simulink model "EBike_Braking"  (R2019b)
settings: Solver=VariableStepAuto  StartTime=0.0  StopTime=1000  MaxStep=0.01  RelTol=1e-3
values from neighbouring files (symbols this model uses):
  A_d = 0.4    [Thesis_Ebike.m]
  Abs = 1    [Thesis_Ebike.m]
  alpha_Conductor = 0.0040    (= 0.004)    [Thesis_Ebike.m]
  Alpha_Magnet = -0.0020    (= -0.002)    [Thesis_Ebike.m]
  Bm = ((Motor_torque_constant)*(17)/(1000*2*pi/60))    (= 0.121753531465)    [Thesis_Ebike.m]
  Braking_Pressure = 100    [Thesis_Ebike.m]
  C_d = 0.9    [Thesis_Ebike.m]
  capacity = 19.5    [Thesis_Ebike.m]
  Coefficient_of_Brake_friction = 0.9    [Thesis_Ebike.m]
  Crank_Length = 0.150    (= 0.15)    [Thesis_Ebike.m]
  Cyclist_weight = 85    [Thesis_Ebike.m]
  Dynamic_Friction_Coefficient = 0.0015    [Thesis_Ebike.m]
  Effective_Radius_of_Disc = 0.16    [Thesis_Ebike.m]
  F_Rider = 100    [Thesis_Ebike.m]
  g = 9.81    [Thesis_Ebike.m]
  Internal_Resistance = 95*10^-3    (= 0.095)    [Thesis_Ebike.m]
  Jm = 10.2 *10^-3    (= 0.0102)    [Thesis_Ebike.m]
  Kb = (51.7/(1000*2*pi/60))    (= 0.493698633471)    [Thesis_Ebike.m]
  L = 0.36*10^-3    (= 0.00036)    [Thesis_Ebike.m]
  Motor_resistance = 88*10^-2    (= 0.88)    [Thesis_Ebike.m]
  Motor_torque_constant = 0.75    [Thesis_Ebike.m]
  Polarization_Capacitance = 1*10^-7    (= 1e-07)    [Thesis_Ebike.m]
  Polarization_Resistance = 95*10^-3    (= 0.095)    [Thesis_Ebike.m]
  Ref_Temp = 25    [Thesis_Ebike.m]
  Rho_air = 1.225    [Thesis_Ebike.m]
  SOC_initial = 100    [Thesis_Ebike.m]
  Static_Friction_Coefficient = 0.0015    [Thesis_Ebike.m]
  Tire_mass = 0.25    [Thesis_Ebike.m]
  Trailer_mass = 50    [Thesis_Ebike.m]
  Vehicle_mass = 25    [Thesis_Ebike.m]
  Wheel_Inertia = 0.0225    [Thesis_Ebike.m]
  Wheel_mass = 0.25    [Thesis_Ebike.m]
  Wheel_Radius = 0.3    [Thesis_Ebike.m]
undefined symbols (not defined in the file or in its folder): sigbuilder_block, V
libraries: simulink x2
(part 1 of 3)
settings Model: Creator=Avmash  LastModifiedBy=Avmash
settings SolverCC: ZeroCrossAlgorithm=Adaptive
settings DebuggingCC: IgnoredZcDiagnostic=none

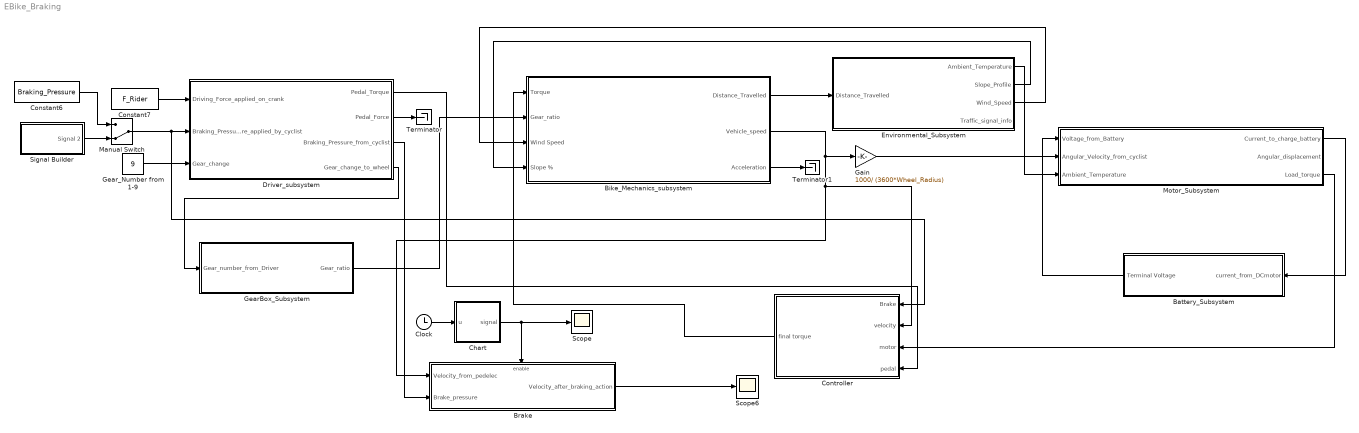
== system EBike_Braking ==
  Battery_Subsystem : Subsystem
  Bike_Mechanics_subsystem : Subsystem
  Brake : Subsystem  TreatAsAtomicUnit=on
  Chart : Stateflow chart  BlockKeywords=__PRM__SERIALIZED__DATA__:Stateflow Chart,Stateflow Diagram  TreatAsAtomicUnit=on
  Clock : Clock
  Constant6 : Constant  Value=Braking_Pressure
  Constant7 : Constant  Value=F_Rider
  Controller : Subsystem
  Driver_subsystem : Subsystem
  Environmental_Subsystem : Subsystem
  Gain : Gain  Gain=1000/ (3600*Wheel_Radius)
  GearBox_Subsystem : Subsystem
  Gear_Number from 1-9 : Constant  Value=9
  Manual Switch : ManualSwitch  CurrentSetting=0
  Motor_Subsystem : Subsystem
  Scope : Scope
  Scope6 : Scope
  Signal Builder : Subsystem  Tag=STV Subsys  LoadFcn=sigbuilder_block('load');  StartFcn=sigbuilder_block('start');  StopFcn=sigbuilder_block('stop');  ClipboardFcn=sigbuilder_block('clipboard');  mask(Sigbuilder block){tuvar=[0:10]}
      mask help: Simulink:masks:SigbuilderBlock_MD
      mask init:
      | if ~strcmp(get_param(bdroot(gcbh),'SimulationStatus'),'stopped') tuvar = sigbuilder_block('maskInit'); end
      settings: CopyFcn=sigbuilder_block('copy');  DeleteFcn=sigbuilder_block('delete');  ModelCloseFcn=sigbuilder_block('modelClose');  PreSaveFcn=sigbuilder_block('preSave');  PauseFcn=sigbuilder_block('pause');  ContinueFcn=sigbuilder_block('continue');  NameChangeFcn=sigbuilder_block('namechange');  OpenFcn=sigbuilder_block('open',[437.6 153 550.4 359.25 ]);  CloseFcn=sigbuilder_block('close');
      mask Display: plot(0, 0, 100, 100,[2, 2, 32, 32, 2], [68, 8, 8, 68, 68],[32, 2], [38, 38], [32, 19, 2],[53, 60, 44], [32, 17, 17, 2],[16, 16, 31, 31]);txt = getActiveGroup(gcbh);text(2, 100, txt,'verticalAlignment', 'top');
  Terminator : Terminator
  Terminator1 : Terminator
  wires:
  Environmental_Subsystem/2(Slope_Profile) -> Bike_Mechanics_subsystem/4(Slope %)
  Environmental_Subsystem/3(Wind_Speed) -> Bike_Mechanics_subsystem/3(Wind Speed)
  Brake/1(Velocity_after_braking_action) -> Scope6/1
  Manual Switch/1 -> Controller/1(Brake), Driver_subsystem/2(Braking_Pressure_applied_by_cyclist)
  Signal Builder/1(Signal 2) -> Manual Switch/2
  Driver_subsystem/3(Braking_Pressure_from_cyclist) -> Brake/2(Brake_pressure)
  Constant6/1 -> Manual Switch/1
  Clock/1 -> Chart/1(u)
  Controller/1("final torque ") -> Bike_Mechanics_subsystem/1(Torque)
  Bike_Mechanics_subsystem/1(Distance_Travelled) -> Environmental_Subsystem/1(Distance_Travelled)
  Chart/1(signal) -> Scope/1, Brake/Enable
  Environmental_Subsystem/1(Ambient_Temperature) -> Motor_Subsystem/3(Ambient_Temperature)
  Gain/1 -> Motor_Subsystem/2(Angular_Velocity_from_cyclist)
  Driver_subsystem/4(Gear_change_to_wheel) -> GearBox_Subsystem/1(Gear_number_from_Driver)
  Bike_Mechanics_subsystem/2(Vehicle_speed) -> Brake/1(Velocity_from_pedelec), Controller/2(velocity), Gain/1
  Motor_Subsystem/1(Current_to_charge_battery) -> Battery_Subsystem/1(current_from_DCmotor)
  Driver_subsystem/1(Pedal_Torque) -> Controller/4(pedal)
  Driver_subsystem/2(Pedal_Force) -> Terminator/1
  GearBox_Subsystem/1(Gear_ratio) -> Bike_Mechanics_subsystem/2(Gear_ratio)
  Constant7/1 -> Driver_subsystem/1(Driving_Force_applied_on_crank)
  Gear_Number from 1-9/1 -> Driver_subsystem/3(Gear_change)
  Motor_Subsystem/3(Load_torque) -> Controller/3(motor)
  Battery_Subsystem/1(Terminal Voltage) -> Motor_Subsystem/1(Voltage_from_Battery)
  Bike_Mechanics_subsystem/3(Acceleration) -> Terminator1/1

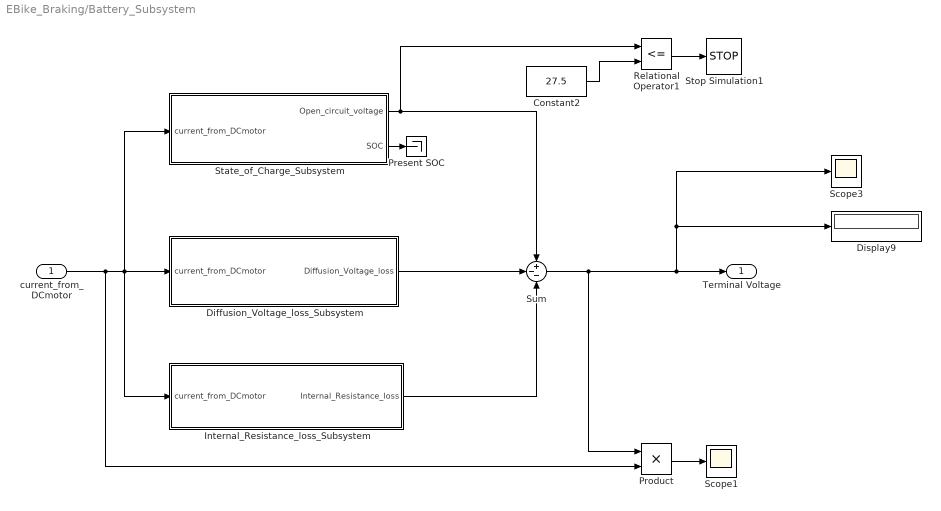
== system EBike_Braking/Battery_Subsystem ==
  current_from_DCmotor : Inport
  Constant2 : Constant  Value=27.5
  Diffusion_Voltage_loss_Subsystem : Subsystem
  Display9 : Display
  Internal_Resistance_loss_Subsystem : Subsystem
  Present SOC : Terminator
  Product : Product
  Relational Operator1 : RelationalOperator  Operator=<=  OutDataTypeStr=boolean  RndMeth=Simplest
  Scope1 : Scope
  Scope3 : Scope
  "State_of_Charge_Subsystem " : Subsystem
  Stop Simulation1 : Stop
  Sum : Sum  Inputs=+--
  Terminal Voltage : Outport  VectorParamsAs1DForOutWhenUnconnected=off
  wires:
  current_from_DCmotor/1 -> Product/2, Internal_Resistance_loss_Subsystem/1(current_from_DCmotor), "State_of_Charge_Subsystem "/1(current_from_DCmotor), Diffusion_Voltage_loss_Subsystem/1(current_from_DCmotor)
  "State_of_Charge_Subsystem "/2(SOC) -> Present SOC/1
  Relational Operator1/1 -> Stop Simulation1/1
  Constant2/1 -> Relational Operator1/2
  Internal_Resistance_loss_Subsystem/1(Internal_Resistance_loss) -> Sum/3
  Diffusion_Voltage_loss_Subsystem/1(Diffusion_Voltage_loss) -> Sum/2
  "State_of_Charge_Subsystem "/1(Open_circuit_voltage) -> Sum/1, Relational Operator1/1
  Sum/1 -> Product/1, Display9/1, Scope3/1, Terminal Voltage/1
  Product/1 -> Scope1/1

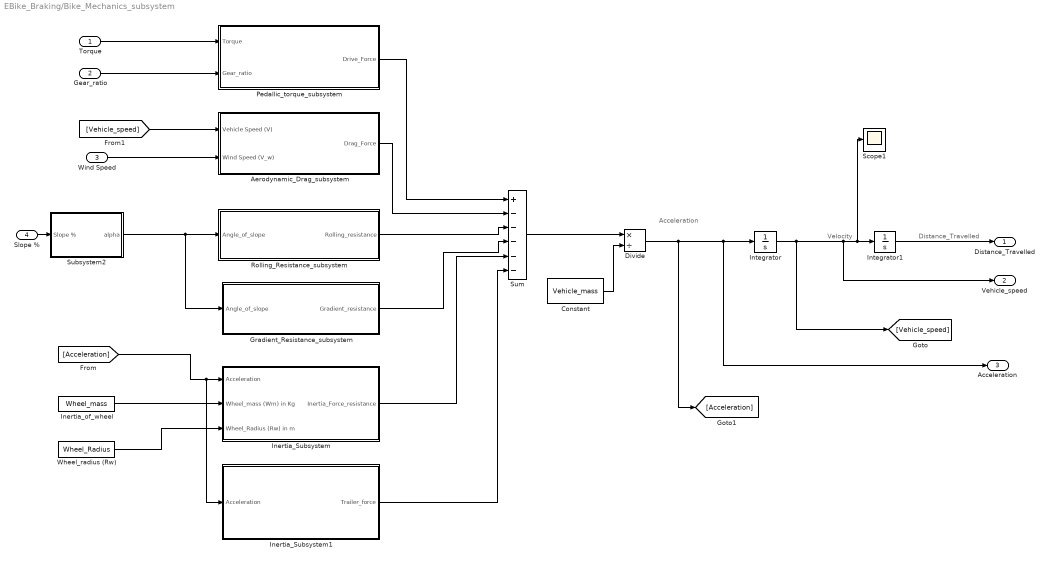
== system EBike_Braking/Bike_Mechanics_subsystem ==
  note: Acceleration
  note: Velocity
  note: Distance_Travelled
  Torque : Inport
  Gear_ratio : Inport  Port=2
  Wind Speed : Inport  Port=3
  Slope % : Inport  Port=4
  Aerodynamic_Drag_subsystem : Subsystem
  Constant : Constant  Value=Vehicle_mass  SampleTime=-1
  Divide : Product  Inputs=*/
  Gradient_Resistance_subsystem : Subsystem
  Inertia_Subsystem : Subsystem
  Inertia_Subsystem1 : Subsystem
  Inertia_of_wheel : Constant  Value=Wheel_mass
  Integrator : Integrator  LowerSaturationLimit=0
  Integrator1 : Integrator
  Pedallic_torque_subsystem : Subsystem
  Rolling_Resistance_subsystem : Subsystem
  Scope1 : Scope
  Subsystem2 : Subsystem
  Sum : Sum  Inputs=+-----
  "Wheel_radius (Rw) " : Constant  Value=Wheel_Radius
  Distance_Travelled : Outport  VectorParamsAs1DForOutWhenUnconnected=off
  Vehicle_speed : Outport  Port=2  VectorParamsAs1DForOutWhenUnconnected=off
  Acceleration : Outport  Port=3  VectorParamsAs1DForOutWhenUnconnected=off
  wires:
  Inertia_Subsystem/1(Inertia_Force_resistance) -> Sum/5
  [Acceleration] -> Inertia_Subsystem1/1(Acceleration), Inertia_Subsystem/1(Acceleration)
  Rolling_Resistance_subsystem/1(Rolling_resistance) -> Sum/3
  "Wheel_radius (Rw) "/1 -> Inertia_Subsystem/3(Wheel_Radius (Rw) in m)
  [Vehicle_speed] -> Aerodynamic_Drag_subsystem/1(Vehicle Speed (V))
  Pedallic_torque_subsystem/1(Drive_Force) -> Sum/1
  Gradient_Resistance_subsystem/1(Gradient_resistance) -> Sum/4
  Wind Speed/1 -> Aerodynamic_Drag_subsystem/2("Wind Speed (V_w) ")
  Aerodynamic_Drag_subsystem/1("Drag_Force ") -> Sum/2
  Inertia_of_wheel/1 -> Inertia_Subsystem/2(Wheel_mass (Wm) in Kg)
  Constant/1 -> Divide/2
  Divide/1 -> Integrator/1, Acceleration/1, [Acceleration]
  Integrator/1 -> [Vehicle_speed], Scope1/1, Integrator1/1, Vehicle_speed/1
  Subsystem2/1(alpha) -> Gradient_Resistance_subsystem/1(Angle_of_slope), Rolling_Resistance_subsystem/1(Angle_of_slope)
  Sum/1 -> Divide/1
  Gear_ratio/1 -> Pedallic_torque_subsystem/2(Gear_ratio)
  Torque/1 -> Pedallic_torque_subsystem/1(Torque)
  Integrator1/1 -> Distance_Travelled/1
  Slope %/1 -> Subsystem2/1(Slope %)
  Inertia_Subsystem1/1(Trailer_force) -> Sum/6

== system EBike_Braking/Brake ==
  Velocity_from_pedelec : Inport
  Brake_pressure : Inport  Port=2
  Enable : EnablePort
  Scope{,1..3} (4 alike) : Scope
  Subsystem1 : Subsystem
  Velocity_after_braking_action : Outport
  wires:
  Subsystem1/2(velocity_of_bike) -> Scope2/1, Velocity_after_braking_action/1
  Velocity_from_pedelec/1 -> Scope/1, Subsystem1/1(velocity)
  Subsystem1/1(Wheel_Velocity) -> Scope1/1
  Subsystem1/3(stopping_distance) -> Scope3/1
  Brake_pressure/1 -> Subsystem1/2(Brake_pressure)

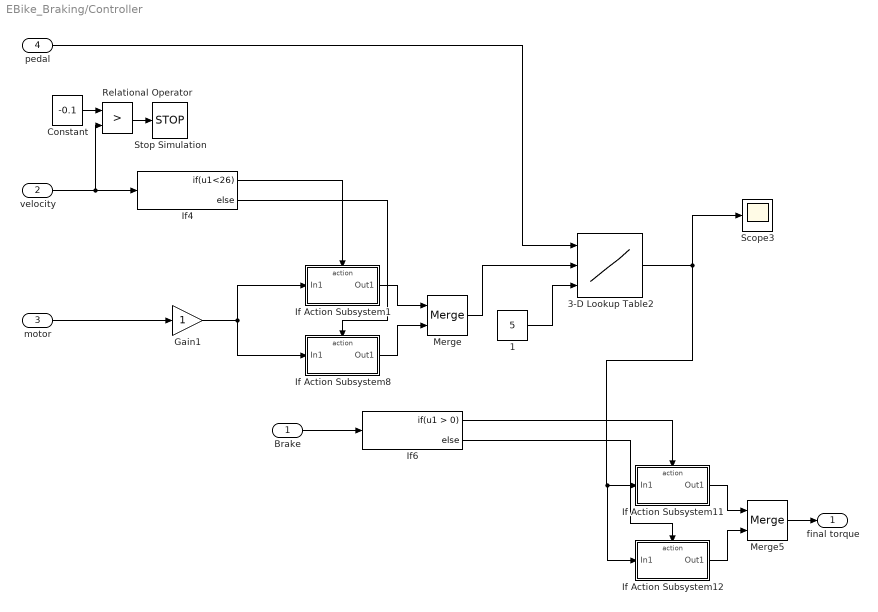
== system EBike_Braking/Controller ==
  Brake : Inport
  velocity : Inport  Port=2
  motor : Inport  Port=3
  pedal : Inport  Port=4
  " 1" : Constant  Value=5
  3-D Lookup Table2 : Lookup_n-D  NumberOfTableDimensions=3  BreakpointsForDimension1=[0,5,10,15,20]  BreakpointsForDimension2=[0,10,20,30,40]  BreakpointsForDimension3=[5, 7]  Table=reshape([0,5,10,15,20,0,10,15,20,25,0,10,20,25,30,0,10,20,30,35,0,10,20,30,40,0,5,10,15,20,0,10,15,20,25,0,10,20,25,30,0,10,20,30,35,0,10,20,30,40],5,5,2)  InternalRulePriority=Speed  RndMeth=Simplest  InputSameDT=on
  Constant : Constant  Value=-0.1
  Gain1 : Gain
  If Action Subsystem1 : Subsystem  TreatAsAtomicUnit=on
  If Action Subsystem11 : Subsystem  TreatAsAtomicUnit=on
  If Action Subsystem12 : Subsystem  TreatAsAtomicUnit=on
  If Action Subsystem8 : Subsystem  TreatAsAtomicUnit=on
  If4 : If  IfExpression=u1<26
  If6 : If
  Merge : Merge
  Merge5 : Merge
  Relational Operator : RelationalOperator  Operator=>  OutDataTypeStr=boolean  RndMeth=Simplest
  Scope3 : Scope
  Stop Simulation : Stop
  "final torque " : Outport
  wires:
  Brake/1 -> If6/1
  If6/2 -> If Action Subsystem12/Action
  If6/1 -> If Action Subsystem11/Action
  If Action Subsystem11/1(Out1) -> Merge5/1
  Merge5/1 -> "final torque "/1
  If Action Subsystem12/1(Out1) -> Merge5/2
  motor/1 -> Gain1/1
  velocity/1 -> Relational Operator/2, If4/1
  " 1"/1 -> 3-D Lookup Table2/3
  If Action Subsystem1/1(Out1) -> Merge/1
  If4/1 -> If Action Subsystem1/Action
  3-D Lookup Table2/1 -> If Action Subsystem12/1(In1), If Action Subsystem11/1(In1), Scope3/1
  Gain1/1 -> If Action Subsystem8/1(In1), If Action Subsystem1/1(In1)
  pedal/1 -> 3-D Lookup Table2/1
  Merge/1 -> 3-D Lookup Table2/2
  If4/2 -> If Action Subsystem8/Action
  If Action Subsystem8/1(Out1) -> Merge/2
  Constant/1 -> Relational Operator/1
  Relational Operator/1 -> Stop Simulation/1

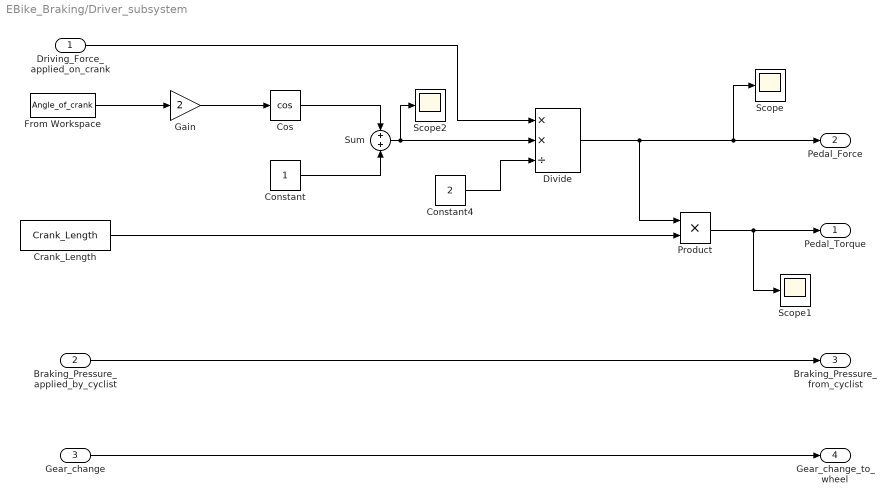
== system EBike_Braking/Driver_subsystem ==
  Driving_Force_applied_on_crank : Inport
  Braking_Pressure_applied_by_cyclist : Inport  Port=2
  Gear_change : Inport  Port=3
  Constant : Constant
  Constant4 : Constant  Value=2
  Cos : Trigonometry  Operator=cos
  Crank_Length : Constant  Value=Crank_Length
  Divide : Product  Inputs=**/
  From Workspace : FromWorkspace  VariableName=Angle_of_crank  SampleTime=0
  Gain : Gain  Gain=2
  Product : Product
  Scope : Scope
  Scope1 : Scope
  Scope2 : Scope
  Sum : Sum
  Pedal_Torque : Outport
  Pedal_Force : Outport  Port=2
  Braking_Pressure_from_cyclist : Outport  Port=3
  Gear_change_to_wheel : Outport  Port=4  VectorParamsAs1DForOutWhenUnconnected=off
  wires:
  Divide/1 -> Scope/1, Pedal_Force/1, Product/1
  Gain/1 -> Cos/1
  Constant/1 -> Sum/2
  Cos/1 -> Sum/1
  Product/1 -> Scope1/1, Pedal_Torque/1
  Constant4/1 -> Divide/3
  Driving_Force_applied_on_crank/1 -> Divide/1
  Sum/1 -> Scope2/1, Divide/2
  Crank_Length/1 -> Product/2
  Braking_Pressure_applied_by_cyclist/1 -> Braking_Pressure_from_cyclist/1
  From Workspace/1 -> Gain/1
  Gear_change/1 -> Gear_change_to_wheel/1

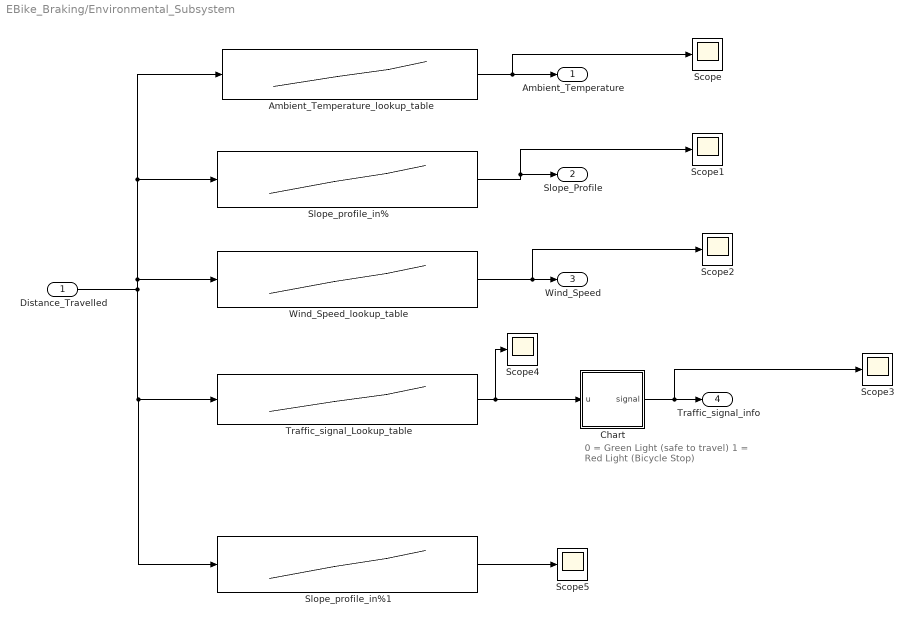
== system EBike_Braking/Environmental_Subsystem ==
  note: 0 = Green Light (safe to travel)
      | 1 = Red Light (Bicycle Stop)
  Distance_Travelled : Inport
  Ambient_Temperature_lookup_table : Lookup_n-D  NumberOfTableDimensions=1  BreakpointsForDimension1=[0 6000 12000]  Table=[25 24 25]  InternalRulePriority=Speed  RndMeth=Simplest  InputSameDT=on
  Chart : Stateflow chart  BlockKeywords=__PRM__SERIALIZED__DATA__:Stateflow Chart,Stateflow Diagram  TreatAsAtomicUnit=on
  Scope{,1..5} (6 alike) : Scope
  Slope_profile_in% : Lookup_n-D  NumberOfTableDimensions=1  BreakpointsForDimension1=|  Table=|  InternalRulePriority=Speed  RndMeth=Simplest  InputSameDT=on
      BreakpointsForDimension1=|
      | [0000,
      | 0015,
      | 0056,
      | 0099,
      | 0108,
      | 0118,
      | 0132,
      | 0142,
      | 0160,
      | 0170,
      | 0186,
      | 0228,
      | 0293,
      | 0336,
      | 0363,
      | 0381,
      | 0391,
      | 0402,
      | 0437,
      | 0478,
      | 0538,
      | 0565,
      | 0582,
      | 0591,
      | 0611,
      | 0640,
      | 0675,
      | 0684,
      | 0699,
      | 0757,
      | 0777,
      | 0788,
      | 0820,
      | 0823,
      | 0837,
      | 0841,
      | 0863,
      | 0880,
      | 0900,
      | 0918,
      | 0948,
      | 0985,
      | 1016,
      | 1037,
      | 1051,
      | 1061,
      | 1082,
      | 1113,
      | 1134,
      | 1142,
      | 1151,
      | 1165,
      | 1176,
      | 1187,
      | 1200,
      | 1216,
      | 1234,
      | 1277,
      | 1341,
      | 1373,
      | 1401,
      | 1452,
      | 1486,
      | 1497,
      | 1507,
      | 1520,
      | 1528,
      | 1557,
      | 1649,
      | 1694,
      | 1716,
      | 1767,
      | 1827,
      | 1898,
      | 1946,
      | 2017,
      | 2030,
      | 2040,
      | 2056,
      | 2110,
      | 2201,
      | 2231,
      | 2242,
      | 2325,
      | 2412,
      | 2504,
      | 2530,
      | 2570,
      | 2607,
      | 2640,
      | 2665,
      | 2713,
      | 2730,
      | 2752,
      | 2763,
      | 2774,
      | 2863,
      | 2961,
      | 3095,
      | 3167,
      | 3268,
      | 3368,
      | 3384,
      | 3418,
      | 3480,
      | 3503,
      | 3562,
      | 3601,
      | 3635,
      | 3719,
      | 3748,
      | 3768,
      | 3844,
      | 3916,
      | 4078,
      | 4224,
      | 4305,
      | 4357,
      | 4398,
      | 4445,
      | 4493,
      | 4548,
      | 4641,
      | 4770,
      | 4916,
      | 5015,
      | 5084,
      | 5110,
      | 5212,
      | 5458,
      | 5491,
      | 5525,
      | 5541,
      | 5551,
      | 5562,
      | 5574,
      | 5591,
      | 5622,
      | 5652,
      | 5665,
      | 5727,
      | 5806,
      | 5856,
      | 5914,
      | 5974,
      | 6031,
      | 6097,
      | 6322,
      | 6482,
      | 6528,
      | 6632,
      | 6688,
      | 6763,
      | 6810,
      | 6853,
      | 6910,
      | 6951,
      | 6998,
      | 7051,
      | 7185,
      | 7248,
      | 7303,
      | 7349,
      | 7386,
      | 7421,
      | 7455,
      | 7492,
      | 7530,
      | 7567,
      | 7609,
      | 7691,
      | 7747,
      | 7751,
      | 7764,
      | 7775,
      | 7808,
      | 7833,
      | 8143,
      | 8170,
      | 8180,
      | 8210,
      | 8811,
      | 8980,
      | 9047,
      | 9065,
      | 9086,
      | 9104,
      | 9141,
      | 9168,
      | 9191,
      | 9215,
      | 9249,
      | 9296,
      | 9348,
      | 9405,
      | 9426,
      | 9442,
      | 9473,
      | 9515,
      | 9550,
      | 9581,
      | 9601,
      | 9627,
      | 9652,
      | 9682,
      | 9735,
      | 9760,
      | 9774,
      | 9784,
      | 9797,
      | 9818,
      | 9838,
      | 9858,
      | 9880,
      | 9972,
      | 10015,
      | 10110,
      | 10128,
      | 10180,
      | 10196,
      | 10262,
      | 10271,
      | 10295,
      | 10311,
      | 10379,
      | 10402,
      | 10421,
      | 10433,
      | 10449,
      | 10470,
      | 10483,
      | 10492,
      | 10501,
      | 10541,
      | 10561,
      | 10573,
      | 10601,
      | 10626,
      | 10652,
      | 10709,
      | 10748,
      | 10809,
      | 10840,
      | 10860,
      | 10877,
      | 10888,
      | 10897,
      | 10912,
      | 10927,
      | 10988,
      | 11013,
      | 11027,
      | 11042,
      | 11084,
      | 11094,
      | 11117,
      | 11138,
      | 11167,
      | 11197,
      | 11251,
      | 11270,
      | 11290,
      | 11304,
      | 11320,
      | 11335,
      | 11351,
      | 11367,
      | 11446,
      | 11492,
      | 11514,
      | 11529,
      | 11540,
      | 11579,
      | 11596,
      | 11645,
      | 11667,
      | 11674,
      | 11689,
      | 11702,
      | 11800
      | ]
      Table=|
      | [0,
      | -0.487804878,
      | -0.23255814,
      | 0,
      | -1,
      | 0,
      | 0,
      | 0,
      | 0,
      | 0,
      | -0.714285714,
      | -0.769230769,
      | -0.697674419,
      | -0.740740741,
      | 0,
      | 0,
      | 0,
      | -0.285714286,
      | -0.243902439,
      | -0.166666667,
      | -0.37037037,
      | -0.588235294,
      | 0,
      | 0,
      | 0,
      | 0,
      | 0,
      | 0,
      | -0.344827586,
      | 0,
      | 0,
      | -0.3125,
      | 0,
      | -0.714285714,
      | 0,
      | 0,
      | 0,
      | 0,
      | 0,
      | 0.333333333,
      | 0.27027027,
      | 0,
      | 0,
      | 0,
      | -1,
      | 0,
      | 0,
      | 0,
      | 0,
      | 0,
      | 0,
      | 0,
      | 0,
      | 0,
      | 0,
      | 0,
      | 0,
      | 0,
      | 0.3125,
      | 0,
      | 0,
      | 0,
      | 0,
      | 0,
      | 0,
      | 0,
      | 0.344827586,
      | 0,
      | 0,
      | 0,
      | 0,
      | 0,
      | 0,
      | 0,
      | 0,
      | 0,
      | 0,
      | 0,
      | -0.185185185,
      | 0,
      | 0,
      | 0,
      | 0,
      | 0,
      | 0,
      | 0,
      | 0,
      | 0,
      | 0,
      | 0,
      | 0,
      | 0.588235294,
      | 0,
      | 0,
      | 0,
      | -0.112359551,
      | 0,
      | 0,
      | 0,
      | 0,
      | 0.1,
      | 0,
      | 0,
      | 0,
      | -0.434782609,
      | -0.169491525,
      | 0,
      | 0,
      | 0,
      | 0,
      | 0,
      | 0,
      | 0,
      | -0.061728395,
      | 0,
      | 0,
      | 0,
      | 0,
      | 0,
      | 0,
      | 0,
      | 0,
      | 0,
      | 0,
      | 0,
      | 0,
      | 0,
      | 0,
      | 0,
      | 0.303030303,
      | 0,
      | 0.625,
      | 0,
      | 0,
      | 0.833333333,
      | 0,
      | 0.322580645,
      | 0,
      | 0,
      | -0.322580645,
      | -0.379746835,
      | 0,
      | 0,
      | 0,
      | 0.175438596,
      | 0,
      | 0,
      | 0,
      | 0,
      | -0.096153846,
      | 0,
      | -0.133333333,
      | 0.212765957,
      | 0,
      | 0,
      | 0,
      | 0.212765957,
      | 0,
      | 0,
      | 0,
      | 0,
      | 0.217391304,
      | 0,
      | 0,
      | 0,
      | 0,
      | 0,
      | 0,
      | 0.238095238,
      | 0.12195122,
      | 0.357142857,
      | 0,
      | 0,
      | 0,
      | 0,
      | 0.4,
      | 0,
      | 0,
      | 0,
      | 0.333333333,
      | 0,
      | 0,
      | 0.149253731,
      | 0,
      | 0,
      | 0,
      | 0,
      | -0.37037037,
      | 0,
      | -0.416666667,
      | 0,
      | -0.212765957,
      | -0.192307692,
      | -0.175438596,
      | 0,
      | 0,
      | 0,
      | -0.238095238,
      | -0.285714286,
      | 0,
      | 0.5,
      | 0.384615385,
      | 0.4,
      | 0,
      | 0,
      | 0,
      | 0,
      | 0,
      | 0,
      | 0,
      | 0,
      | 0,
      | 0,
      | 0,
      | 0,
      | 0,
      | 0,
      | 0.192307692,
      | 0,
      | 0,
      | 0,
      | 0,
      | 0,
      | 0,
      | 0,
      | 0,
      | 0,
      | 0,
      | 0,
      | 0,
      | 0,
      | 0,
      | 0,
      | 0.5,
      | 0,
      | 0,
      | 0,
      | 0,
      | 0,
      | 0,
      | 0,
      | 0,
      | 0,
      | -0.588235294,
      | 0,
      | 0,
      | 0,
      | 0,
      | 0,
      | 0,
      | 0,
      | 0,
      | 0,
      | 0,
      | 0,
      | 0,
      | 0,
      | 0,
      | 0,
      | 0,
      | 0,
      | 0,
      | 0.625,
      | 0,
      | 0,
      | 0,
      | -0.126582278,
      | 0,
      | 0,
      | 0,
      | 0,
      | 0,
      | 0,
      | 0,
      | 0,
      | 0,
      | 0,
      | 0,
      | 0,
      | 0,
      | ]
  Slope_profile_in%1 : Lookup_n-D  NumberOfTableDimensions=1  BreakpointsForDimension1=|  IndexSearchMethod=Linear search  Table=|  InternalRulePriority=Speed  RndMeth=Simplest  InputSameDT=on
      BreakpointsForDimension1=|
      | [0000,
      | 0015,
      | 0056,
      | 0099,
      | 0108,
      | 0118,
      | 0132,
      | 0142,
      | 0160,
      | 0170,
      | 0186,
      | 0228,
      | 0293,
      | 0336,
      | 0363,
      | 0381,
      | 0391,
      | 0402,
      | 0437,
      | 0478,
      | 0538,
      | 0565,
      | 0582,
      | 0591,
      | 0611,
      | 0640,
      | 0675,
      | 0684,
      | 0699,
      | 0757,
      | 0777,
      | 0788,
      | 0820,
      | 0823,
      | 0837,
      | 0841,
      | 0863,
      | 0880,
      | 0900,
      | 0918,
      | 0948,
      | 0985,
      | 1016,
      | 1037,
      | 1051,
      | 1061,
      | 1082,
      | 1113,
      | 1134,
      | 1142,
      | 1151,
      | 1165,
      | 1176,
      | 1187,
      | 1200,
      | 1216,
      | 1234,
      | 1277,
      | 1341,
      | 1373,
      | 1401,
      | 1452,
      | 1486,
      | 1497,
      | 1507,
      | 1520,
      | 1528,
      | 1557,
      | 1649,
      | 1694,
      | 1716,
      | 1767,
      | 1827,
      | 1898,
      | 1946,
      | 2017,
      | 2030,
      | 2040,
      | 2056,
      | 2110,
      | 2201,
      | 2231,
      | 2242,
      | 2325,
      | 2412,
      | 2504,
      | 2530,
      | 2570,
      | 2607,
      | 2640,
      | 2665,
      | 2713,
      | 2730,
      | 2752,
      | 2763,
      | 2774,
      | 2863,
      | 2961,
      | 3095,
      | 3167,
      | 3268,
      | 3368,
      | 3384,
      | 3418,
      | 3480,
      | 3503,
      | 3562,
      | 3601,
      | 3635,
      | 3719,
      | 3748,
      | 3768,
      | 3844,
      | 3916,
      | 4078,
      | 4224,
      | 4305,
      | 4357,
      | 4398,
      | 4445,
      | 4493,
      | 4548,
      | 4641,
      | 4770,
      | 4916,
      | 5015,
      | 5084,
      | 5110,
      | 5212,
      | 5458,
      | 5491,
      | 5525,
      | 5541,
      | 5551,
      | 5562,
      | 5574,
      | 5591,
      | 5622,
      | 5652,
      | 5665,
      | 5727,
      | 5806,
      | 5856,
      | 5914,
      | 5974,
      | 6031,
      | 6097,
      | 6322,
      | 6482,
      | 6528,
      | 6632,
      | 6688,
      | 6763,
      | 6810,
      | 6853,
      | 6910,
      | 6951,
      | 6998,
      | 7051,
      | 7185,
      | 7248,
      | 7303,
      | 7349,
      | 7386,
      | 7421,
      | 7455,
      | 7492,
      | 7530,
      | 7567,
      | 7609,
      | 7691,
      | 7747,
      | 7751,
      | 7764,
      | 7775,
      | 7808,
      | 7833,
      | 8143,
      | 8170,
      | 8180,
      | 8210,
      | 8811,
      | 8980,
      | 9047,
      | 9065,
      | 9086,
      | 9104,
      | 9141,
      | 9168,
      | 9191,
      | 9215,
      | 9249,
      | 9296,
      | 9348,
      | 9405,
      | 9426,
      | 9442,
      | 9473,
      | 9515,
      | 9550,
      | 9581,
      | 9601,
      | 9627,
      | 9652,
      | 9682,
      | 9735,
      | 9760,
      | 9774,
      | 9784,
      | 9797,
      | 9818,
      | 9838,
      | 9858,
      | 9880,
      | 9972,
      | 10015,
      | 10110,
      | 10128,
      | 10180,
      | 10196,
      | 10262,
      | 10271,
      | 10295,
      | 10311,
      | 10379,
      | 10402,
      | 10421,
      | 10433,
      | 10449,
      | 10470,
      | 10483,
      | 10492,
      | 10501,
      | 10541,
      | 10561,
      | 10573,
      | 10601,
      | 10626,
      | 10652,
      | 10709,
      | 10748,
      | 10809,
      | 10840,
      | 10860,
      | 10877,
      | 10888,
      | 10897,
      | 10912,
      | 10927,
      | 10988,
      | 11013,
      | 11027,
      | 11042,
      | 11084,
      | 11094,
      | 11117,
      | 11138,
      | 11167,
      | 11197,
      | 11251,
      | 11270,
      | 11290,
      | 11304,
      | 11320,
      | 11335,
      | 11351,
      | 11367,
      | 11446,
      | 11492,
      | 11514,
      | 11529,
      | 11540,
      | 11579,
      | 11596,
      | 11645,
      | 11667,
      | 11674,
      | 11689,
      | 11702,
      | 11800
      | ]
      Table=|
      | [39,
      | 39,
      | 37,
      | 36,
      | 36,
      | 35,
      | 35,
      | 35,
      | 35,
      | 35,
      | 35,
      | 32,
      | 27,
      | 24,
      | 22,
      | 22,
      | 22,
      | 22,
      | 21,
      | 20,
      | 19,
      | 18,
      | 17,
      | 17,
      | 17,
      | 17,
      | 17,
      | 17,
      | 17,
      | 15,
      | 15,
      | 15,
      | 14,
      | 14,
      | 13,
      | 13,
      | 13,
      | 13,
      | 13,
      | 13,
      | 14,
      | 15,
      | 15,
      | 15,
      | 15,
      | 14,
      | 14,
      | 14,
      | 14,
      | 14,
      | 14,
      | 14,
      | 14,
      | 14,
      | 14,
      | 14,
      | 14,
      | 14,
      | 14,
      | 15,
      | 15,
      | 15,
      | 15,
      | 15,
      | 15,
      | 15,
      | 15,
      | 16,
      | 16,
      | 16,
      | 16,
      | 16,
      | 16,
      | 16,
      | 16,
      | 16,
      | 16,
      | 16,
      | 16,
      | 15,
      | 15,
      | 15,
      | 15,
      | 15,
      | 15,
      | 15,
      | 15,
      | 15,
      | 15,
      | 15,
      | 15,
      | 15,
      | 16,
      | 16,
      | 16,
      | 16,
      | 15,
      | 15,
      | 15,
      | 15,
      | 15,
      | 16,
      | 16,
      | 16,
      | 16,
      | 15,
      | 14,
      | 14,
      | 14,
      | 14,
      | 14,
      | 14,
      | 14,
      | 14,
      | 13,
      | 13,
      | 13,
      | 13,
      | 13,
      | 13,
      | 13,
      | 13,
      | 13,
      | 13,
      | 13,
      | 13,
      | 13,
      | 13,
      | 13,
      | 13,
      | 14,
      | 14,
      | 15,
      | 15,
      | 15,
      | 16,
      | 16,
      | 17,
      | 17,
      | 17,
      | 15,
      | 12,
      | 12,
      | 12,
      | 12,
      | 13,
      | 13,
      | 13,
      | 13,
      | 13,
      | 12,
      | 12,
      | 11,
      | 12,
      | 12,
      | 12,
      | 12,
      | 13,
      | 13,
      | 13,
      | 13,
      | 13,
      | 14,
      | 14,
      | 14,
      | 14,
      | 14,
      | 14,
      | 14,
      | 15,
      | 16,
      | 18,
      | 18,
      | 18,
      | 18,
      | 18,
      | 19,
      | 19,
      | 19,
      | 19,
      | 20,
      | 20,
      | 20,
      | 21,
      | 21,
      | 21,
      | 21,
      | 21,
      | 20,
      | 20,
      | 19,
      | 19,
      | 18,
      | 17,
      | 16,
      | 16,
      | 16,
      | 16,
      | 15,
      | 14,
      | 14,
      | 15,
      | 16,
      | 17,
      | 17,
      | 17,
      | 17,
      | 17,
      | 17,
      | 17,
      | 17,
      | 17,
      | 17,
      | 17,
      | 17,
      | 17,
      | 17,
      | 17,
      | 18,
      | 18,
      | 18,
      | 18,
      | 18,
      | 18,
      | 18,
      | 18,
      | 18,
      | 18,
      | 18,
      | 18,
      | 18,
      | 18,
      | 18,
      | 18,
      | 19,
      | 19,
      | 19,
      | 19,
      | 19,
      | 19,
      | 19,
      | 19,
      | 19,
      | 19,
      | 18,
      | 18,
      | 18,
      | 18,
      | 18,
      | 18,
      | 18,
      | 18,
      | 18,
      | 18,
      | 18,
      | 18,
      | 18,
      | 18,
      | 18,
      | 18,
      | 18,
      | 18,
      | 18,
      | 19,
      | 19,
      | 19,
      | 19,
      | 18,
      | 18,
      | 18,
      | 18,
      | 18,
      | 18,
      | 18,
      | 18,
      | 18,
      | 18,
      | 18,
      | 18,
      | 18
      | ]
  Traffic_signal_Lookup_table : Lookup_n-D  NumberOfTableDimensions=1  BreakpointsForDimension1=|  Table=|  InternalRulePriority=Speed  RndMeth=Simplest  InputSameDT=on
      BreakpointsForDimension1=|
      | [0,
      | 1352.604,
      | 1352.624,
      | 1352.644,
      | 2594.125,
      | 2594.145,
      | 2594.165,
      | 5283.812,
      | 5283.832,
      | 5283.852,
      | 7423.782,
      | 7423.802,
      | 7423.822,
      | 9090.133,
      | 9090.153,
      | 9090.173,
      | 9442.834,
      | 9442.854,
      | 9442.874,
      | 9911.784,
      | 9911.804,
      | 9911.824,
      | 10337.11,
      | 10337.31,
      | 10337.51,
      | 10698.74,
      | 10698.94,
      | 10699.14,
      | 11070.92,
      | 11071.12,
      | 11071.32,
      | 11082.84,
      | 11083.04,
      | 11083.24,
      | 11800
      | ]
      Table=|
      | [
      | 0,
      | 0,
      | 1,
      | 0,
      | 0,
      | 1,
      | 0,
      | 0,
      | 1,
      | 0,
      | 0,
      | 1,
      | 0,
      | 0,
      | 1,
      | 0,
      | 0,
      | 1,
      | 0,
      | 0,
      | 1,
      | 0,
      | 0,
      | 1,
      | 0,
      | 0,
      | 1,
      | 0,
      | 0,
      | 1,
      | 0,
      | 0,
      | 1,
      | 0,
      | 0]
  Wind_Speed_lookup_table : Lookup_n-D  NumberOfTableDimensions=1  BreakpointsForDimension1=[0 5999.9 6000 12000]  Table=[0 0 0 0]  InternalRulePriority=Speed  RndMeth=Simplest  InputSameDT=on
  Ambient_Temperature : Outport  VectorParamsAs1DForOutWhenUnconnected=off
  Slope_Profile : Outport  Port=2  VectorParamsAs1DForOutWhenUnconnected=off
  Wind_Speed : Outport  Port=3  VectorParamsAs1DForOutWhenUnconnected=off
  Traffic_signal_info : Outport  Port=4  VectorParamsAs1DForOutWhenUnconnected=off
  wires:
  Distance_Travelled/1 -> Ambient_Temperature_lookup_table/1, Slope_profile_in%/1, Wind_Speed_lookup_table/1, Slope_profile_in%1/1, Traffic_signal_Lookup_table/1
  Wind_Speed_lookup_table/1 -> Scope2/1, Wind_Speed/1
  Ambient_Temperature_lookup_table/1 -> Ambient_Temperature/1, Scope/1
  Slope_profile_in%/1 -> Slope_Profile/1, Scope1/1
  Chart/1(signal) -> Scope3/1, Traffic_signal_info/1
  Traffic_signal_Lookup_table/1 -> Chart/1(u), Scope4/1
  Slope_profile_in%1/1 -> Scope5/1

== system EBike_Braking/GearBox_Subsystem ==
  Gear_number_from_Driver : Inport
  Crankset_Teeth : Constant  Value=34
  Divide : Product  Inputs=*/
  Gear_Box_Subsystem : Subsystem
  Gear_ratio : Outport  VectorParamsAs1DForOutWhenUnconnected=off
  wires:
  Divide/1 -> Gear_ratio/1
  Gear_number_from_Driver/1 -> Gear_Box_Subsystem/1(Gear_Number)
  Gear_Box_Subsystem/1(Final_Gear_Teeth) -> Divide/1
  Crankset_Teeth/1 -> Divide/2

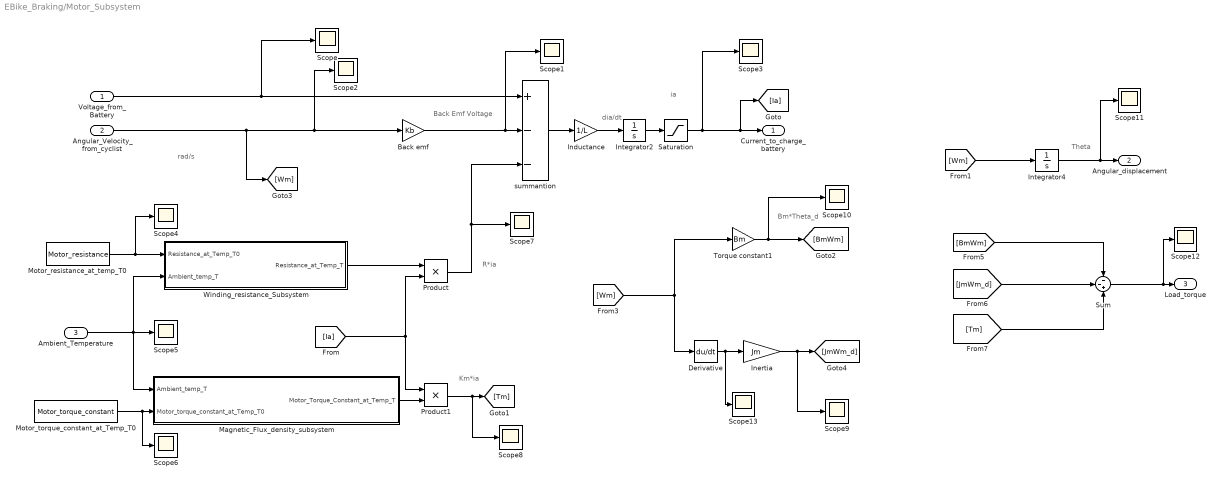
== system EBike_Braking/Motor_Subsystem ==
  note: ia
  note: dia/dt
  note: rad/s
  note: R*ia
  note: Km*ia
  note: Theta
  note: Bm*Theta_d
  note: Back Emf Voltage
  Voltage_from_Battery : Inport
  Angular_Velocity_from_cyclist : Inport  Port=2
  Ambient_Temperature : Inport  Port=3
  Back emf : Gain  Gain=Kb
  Derivative : Derivative
  Inductance : Gain  Gain=1/L
  Inertia : Gain  Gain=Jm
  Integrator2 : Integrator
  Integrator4 : Integrator
  Magnetic_Flux_density_subsystem : Subsystem
  Motor_resistance_at_temp_T0 : Constant  Value=Motor_resistance  SampleTime=-1
  Motor_torque_constant_at_Temp_T0 : Constant  Value=Motor_torque_constant  SampleTime=-1
  Product : Product
  Product1 : Product
  Saturation : Saturate  UpperLimit=inf  LowerLimit=-inf
  Scope{,1..13} (14 alike) : Scope
  Sum : Sum  Inputs=--+
  Torque constant1 : Gain  Gain=Bm
  Winding_resistance_Subsystem : Subsystem
  summantion : Sum  Inputs=+--
  Current_to_charge_battery : Outport  VectorParamsAs1DForOutWhenUnconnected=off
  Angular_displacement : Outport  Port=2  VectorParamsAs1DForOutWhenUnconnected=off
  Load_torque : Outport  Port=3
  wires:
  Back emf/1 -> Scope1/1, summantion/2
  Inductance/1 -> Integrator2/1
  summantion/1 -> Inductance/1
  [Wm] -> Integrator4/1
  Motor_resistance_at_temp_T0/1 -> Scope4/1, Winding_resistance_Subsystem/1(Resistance_at_Temp_T0)
  Product/1 -> summantion/3, Scope7/1
  Ambient_Temperature/1 -> Winding_resistance_Subsystem/2(Ambient_temp_T), Scope5/1, Magnetic_Flux_density_subsystem/1(Ambient_temp_T)
  Motor_torque_constant_at_Temp_T0/1 -> Scope6/1, Magnetic_Flux_density_subsystem/2(Motor_torque_constant_at_Temp_T0)
  [Ia] -> Product1/1, Product/2
  Magnetic_Flux_density_subsystem/1(Motor_Torque_Constant_at_Temp_T) -> Product1/2
  Torque constant1/1 -> Scope10/1, [BmWm]
  Product1/1 -> Scope8/1, [Tm]
  Integrator4/1 -> Scope11/1, Angular_displacement/1
  Winding_resistance_Subsystem/1(Resistance_at_Temp_T) -> Product/1
  Angular_Velocity_from_cyclist/1 -> [Wm], Scope2/1, Back emf/1
  [Wm] -> Torque constant1/1, Derivative/1
  Derivative/1 -> Scope13/1, Inertia/1
  Inertia/1 -> Scope9/1, [JmWm_d]
  [Tm] -> Sum/3
  [JmWm_d] -> Sum/2
  [BmWm] -> Sum/1
  Voltage_from_Battery/1 -> Scope/1, summantion/1
  Sum/1 -> Scope12/1, Load_torque/1
  Integrator2/1 -> Saturation/1
  Saturation/1 -> Scope3/1, [Ia], Current_to_charge_battery/1

== system EBike_Braking/Signal Builder ==
  Demux : Demux  Tag=STV Demux  Outputs=1
  FromWs : FromWorkspace  Tag=STV FromWs  VariableName=tuvar  SampleTime=0
      SigBuilderData=|
      | common.afterFinalStr = 'Extrapolate'
      | common.sampleTime = 0
      | dataSet.timeRange = [0 1000]
      | dataSet.name = 'Group 1'
      | sbobj.Groups.Name = 'Group 1'
      | sbobj.Groups.Signals.Name = 'Signal 2'
      | sbobj.Groups.Signals.XData = [0 500 500 1000]
      | sbobj.Groups.Signals.YData = [0 0 200 200]
      | sbobj.Groups.TimeRange = [0 1000]
  Signal 2 : Outport  Tag=STV Outport
  wires:
  FromWs/1 -> Demux/1
  Demux/1 -> Signal 2/1

== system EBike_Braking/Battery_Subsystem/Diffusion_Voltage_loss_Subsystem ==
  current_from_DCmotor : Inport
  1RC Setup : Gain
  Constant2 : Constant  Value=Polarization_Capacitance  SampleTime=-1
  Constant3 : Constant  Value=Polarization_Resistance  SampleTime=-1
  Divide : Product  Inputs=*/
  Divide1 : Product  Inputs=/*
  Integrator : Integrator
  Product : Product
  Scope3 : Scope
  Sum1 : Sum  Inputs=+|-
  Diffusion_Voltage_loss : Outport  VectorParamsAs1DForOutWhenUnconnected=off
  wires:
  Divide/1 -> Sum1/1
  Integrator/1 -> 1RC Setup/1
  Divide1/1 -> Sum1/2
  Constant3/1 -> Product/2
  Product/1 -> Divide1/1
  Sum1/1 -> Integrator/1
  current_from_DCmotor/1 -> Divide/1
  Constant2/1 -> Product/1, Divide/2
  1RC Setup/1 -> Scope3/1, Diffusion_Voltage_loss/1, Divide1/2

== system EBike_Braking/Battery_Subsystem/Internal_Resistance_loss_Subsystem ==
  current_from_DCmotor : Inport
  Constant : Constant  Value=Internal_Resistance  SampleTime=-1
  Product1 : Product
  Scope : Scope
  Internal_Resistance_loss : Outport  VectorParamsAs1DForOutWhenUnconnected=off
  wires:
  current_from_DCmotor/1 -> Product1/1
  Constant/1 -> Product1/2
  Product1/1 -> Scope/1, Internal_Resistance_loss/1
